simulink model "mimaquina"  (R2013a)
settings: Solver=ode45  StartTime=0.0  StopTime=50  RelTol=1e-3
values from neighbouring files (symbols this model uses):
  I1 = .004    (= 0.004)    [miosinlazoalgebraico.m]    (also in yovalores.m = 1)
  I2 = .005    (= 0.005)    [miosinlazoalgebraico.m]    (also in yovalores.m = 1)
  phi1 = m2*lc2*lc2    (= 0.028158)    [yovalores.m]
  phi2 = l1*lc2*m2    (= 0.063726)    [yovalores.m]
  phi3 = m1*g*lc1    (= 1.5396795)    [yovalores.m]
  phi4 = m2*g*lc2    (= 1.453842)    [yovalores.m]
  phi5 = m2*g*l1    (= 3.290274)    [yovalores.m]
  phi6 = m2*l1*l1    (= 0.144222)    [yovalores.m]
  phi7 = m1*lc1*lc1    (= 0.03374425)    [yovalores.m]
settings Model: Creator=Daniel  LastModifiedBy=Daniel

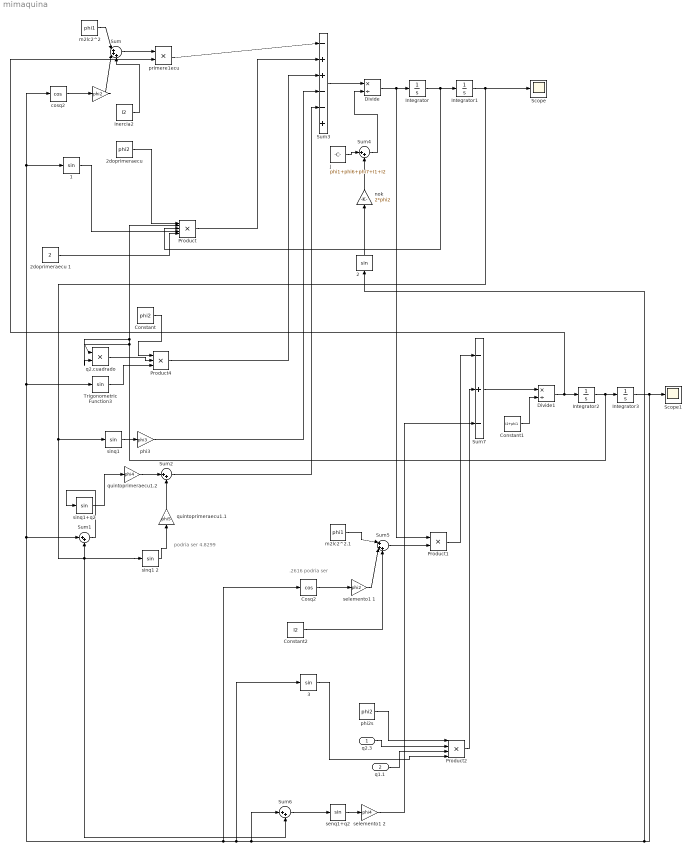
== system mimaquina ==
  note: podria ser 4.8299
  note: .2616 podria ser
  q2.3 : Inport
  q1.1 : Inport  Port=2
  " " : Gain  Gain=phi2
  " nok " : Gain  Gain=2*phi2
  " 1" : Trigonometry
  " 2" : Trigonometry
  " 3" : Trigonometry
  "2doprimeraecu " : Constant  Value=phi2
  2doprimeraecu 1 : Constant  Value=2
  Constant : Constant  Value=phi2
  Constant1 : Constant  Value=I2+phi1
  Constant2 : Constant  Value=I2
  Cosq2 : Trigonometry  Operator=cos
  Divide : Product  Inputs=*/
  Divide1 : Product  Inputs=*/
  Inercia2 : Constant  Value=I2
  Integrator : Integrator
  Integrator1 : Integrator  InitialCondition=pi
  Integrator2 : Integrator
  Integrator3 : Integrator  InitialCondition=pi
  J : Constant  Value=phi1+phi6+phi7+I1+I2
  Product : Product  Inputs=5
  Product1 : Product
  Product2 : Product  Inputs=4
  Product4 : Product  Inputs=3
  Scope : Scope
      settings: YMin=-5300  YMax=-4925
  Scope1 : Scope
      settings: YMin=-2.9565  YMax=-2.948
  Sum : Sum  Inputs=|+++
  Sum{1..2,4,6} (4 alike) : Sum  Inputs=|++
  Sum3 : Sum  Inputs=|-++--+
  Sum5 : Sum  Inputs=|+++
  Sum7 : Sum  Inputs=|-+-
  Trigonometric Function3 : Trigonometry
  cosq2 : Trigonometry  Operator=cos
  m2lc2^2 : Constant  Value=phi1
  m2lc2^2.1 : Constant  Value=phi1
  "phi2s " : Constant  Value=phi2
  phi3 : Gain  Gain=phi3  LockScale=on
  primere1ecu : Product
  q2.cuadrado : Product
  quintoprimeraecu1.1 : Gain  Gain=phi5  LockScale=on
  quintoprimeraecu1.2 : Gain  Gain=phi4  LockScale=on
  selemento1 1 : Gain  Gain=phi2
  selemento1 2 : Gain  Gain=phi4
  senq1+q2 : Trigonometry
  "sinq1 " : Trigonometry
  sinq1 2 : Trigonometry
  "sinq1+q2 " : Trigonometry
  wires:
  m2lc2^2/1 -> Sum/1
  cosq2/1 -> " "/1
  " "/1 -> Sum/2
  Sum/1 -> primere1ecu/1
  Divide1/1 -> primere1ecu/2, Integrator2/1
  Inercia2/1 -> Sum/3
  Integrator3/1 -> Trigonometric Function3/1, cosq2/1, " 1"/1, Sum1/1, Cosq2/1, " 3"/1, Sum6/1, " 2"/1, Scope1/1
  " 1"/1 -> Product/4
  "2doprimeraecu "/1 -> Product/1
  Integrator/1 -> Product/3, Integrator1/1
  2doprimeraecu 1/1 -> Product/5
  Integrator2/1 -> q2.cuadrado/1, q2.cuadrado/2, Product/2, Integrator3/1
  q2.cuadrado/1 -> Product4/2
  Trigonometric Function3/1 -> Product4/3
  Constant/1 -> Product4/1
  "sinq1 "/1 -> phi3/1
  "sinq1+q2 "/1 -> quintoprimeraecu1.2/1
  quintoprimeraecu1.2/1 -> Sum2/1
  Sum1/1 -> "sinq1+q2 "/1
  Integrator1/1 -> "sinq1 "/1, sinq1 2/1, Sum1/2, Sum6/2, Scope/1
  sinq1 2/1 -> quintoprimeraecu1.1/1
  quintoprimeraecu1.1/1 -> Sum2/2
  Sum2/1 -> Sum3/5
  Sum3/1 -> Divide/1
  primere1ecu/1 -> Sum3/1
  Product/1 -> Sum3/2
  Product4/1 -> Sum3/3
  phi3/1 -> Sum3/4
  J/1 -> Sum4/1
  " nok "/1 -> Sum4/2
  " 2"/1 -> " nok "/1
  Sum4/1 -> Divide/2
  Cosq2/1 -> selemento1 1/1
  selemento1 1/1 -> Sum5/2
  m2lc2^2.1/1 -> Sum5/1
  Product1/1 -> Sum7/1
  Sum5/1 -> Product1/2
  Divide/1 -> Product1/1, Integrator/1
  Constant2/1 -> Sum5/3
  q1.1/1 -> Product2/3
  q2.3/1 -> Product2/2
  " 3"/1 -> Product2/4
  "phi2s "/1 -> Product2/1
  Product2/1 -> Sum7/2
  selemento1 2/1 -> Sum7/3
  Sum6/1 -> senq1+q2/1
  senq1+q2/1 -> selemento1 2/1
  Sum7/1 -> Divide1/1
  Constant1/1 -> Divide1/2
